simulink model "PMSM_Model"  (R2024b)
settings: Solver=FixedStepAuto  StartTime=0.0  StopTime=3  FixedStep=1e-5  MaxStep=1e-4  RelTol=1e-4
model workspace: external: MAT-File D:\EV\Graduation_project\Motor_Model_mathmatical\Model_Calculations.mat (data not in the file)
undefined symbols (not defined in the file): B, f, J, Ki_d, Ki_q, Ki_s, Kp_q, Kp_s, lambda, lamdaM, Ld, Ls, p, P, R, Rs, Tc, Vm
libraries: simulink x3, eeStairGenerator x1
settings Model: Creator=ahmed  LastModifiedBy=ahmed
settings SolverCC: ZeroCrossAlgorithm=Adaptive
settings DebuggingCC: ConsistencyChecking=warning  IgnoredZcDiagnostic=none

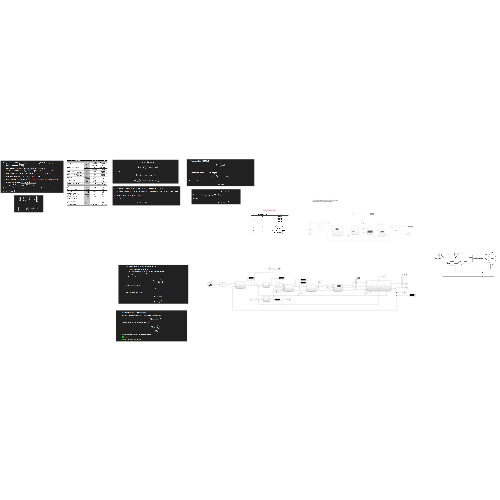
[thumbnail: Simulink's stored preview of the top-level diagram]
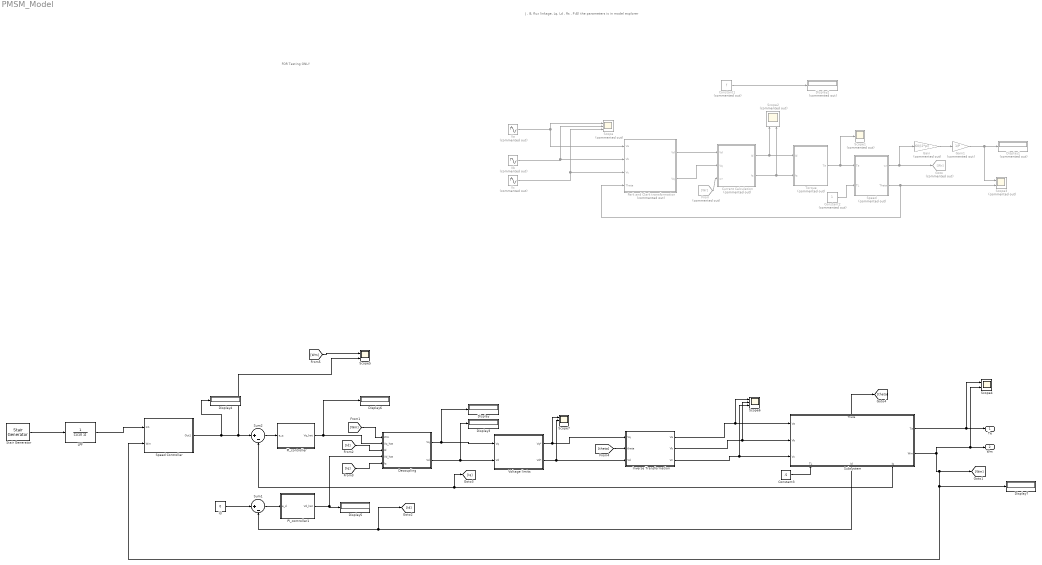
== system PMSM_Model ==
  note: FOR Testing ONLY
  note: J , B, flux linkage, Lq, Ld , Rs , P All the parameters is in model explorer
  Constant1 : Constant  Commented=on  Value=f
  Constant2 : Constant  Commented=on
  Constant3 : Constant  Value=.5
  Current Calculation : Subsystem  Commented=on
  "Decoupling " : Subsystem
  Display{,3..7} (6 alike) : Display
  Display1 : Display  Commented=on
  Display2 : Display  Commented=on
  From : From  Commented=on  GotoTag=Wr
  Gain : Gain  Commented=on  Gain=60/(2*pi)
  Gain1 : Gain  Commented=on  Gain=1/P
  Goto : Goto  Commented=on  GotoTag=Wr
  Id : Constant  Value=0
  Inverse Transformation : Subsystem
  LPF : TransferFcn  Denominator=[1/10 1]
  PI_controller : Subsystem
  PI_controller1 : Subsystem
  Park and Clark transformation : Subsystem  Commented=on
  Scope : Scope  Commented=on  NumInputPorts=3
  Scope1 : Scope  Commented=on
  Scope2 : Scope  Commented=on  NumInputPorts=2
  Scope3 : Scope  Commented=on  NumInputPorts=2
  Scope4 : Scope  NumInputPorts=2
  Scope5 : Scope  NumInputPorts=2
  Scope6 : Scope  NumInputPorts=3
  Scope7 : Scope  NumInputPorts=3
  Speed : Subsystem  Commented=on
  "Speed Controller " : Subsystem
  Stair Generator : eeStairGenerator/Stair Generator  LabelModeActiveChoice=Discrete  TimeInput=[0 1 1.3 1.7 2 2.4]  AmplitudeInput=[200 1000 3000 4500 2000 0]  SampleTime=1e-5  RepeatPattern=off  OutDataTypeStr=double
      settings: LibrarySourceBlock=ee_sl_lib/General Control/Stair Generator
  Subsystem : Subsystem
      settings: PortSchema="{\"entries\":[{\"content\":{\"sides\":[{\"content\":{\"connectorIds\":[\"In1\",\"In2\",\"In3\"]},\"type\":\"ConnectorPlacement.EquallySpacedRectSide\",\"uuid\":\"410fafe1-6d3d-4b62-9ccb-454f6008b81a\"},{\"content\":{\"connectorIds\":[\"Out1\",\"Out2\"],\"side\":\"RIGHT\"},\"type\":\"ConnectorPlacement.EquallySpacedRectSide\",\"uuid\":\"b4215a85-6f2a-4bbd-a305-1fa3c25faaac\"},{\"content\":{\"connectorIds\":[\"Out5\"],\"side\":\"TOP\"},\"type\":\"ConnectorPlacement.EquallySpacedRectSide\",\"uuid\":\"c3471a58-e27d-4fa8-ab5e-4301d929309b\"},{\"content\":{\"connectorIds\":[\"In4\",\"Out3\",\"Out4\"],\"side\":\"BOTTOM\"},\"type\":\"ConnectorPlacement.EquallySpacedRectSide\",\"uuid\":\"92e7eecc-1ce6-457d-b998-008a2505e29d\"}]},\"type\":\"ConnectorPlacement.EquallySpacedConnector\",\"uuid\":\"8b1e994c-6614-4fb4-bf28-22b9fb88c59f\"}],\"packageUris\":[\"http://schema.mathworks.com/mf0/Connector/R2020b\"],\"version\":\"1.0\"}"
  Sum1 : Sum  Inputs=|+-
  Sum2 : Sum  Inputs=|+-
  "Torque " : Subsystem  Commented=on
  Va : Sin  Commented=on  Amplitude=Vm  Frequency=2*f*pi  SampleTime=0
  Vb : Sin  Commented=on  Amplitude=Vm  Frequency=2*f*pi  Phase=-(120*(pi/180))  SampleTime=0
  Vc : Sin  Commented=on  Amplitude=Vm  Frequency=2*f*pi  Phase=-(240*(pi/180))  SampleTime=0
  Voltage limits : Subsystem
  Te : Outport
  Wm : Outport  Port=2
  wires:
  Va/1 -> Park and Clark transformation/1(Va), Scope/1
  Vb/1 -> Scope/2, Park and Clark transformation/2(Vb)
  Vc/1 -> Scope/3, Park and Clark transformation/3(Vc)
  Park and Clark transformation/1(Vd) -> Current Calculation/1(Vd)
  Park and Clark transformation/2(Vq) -> Current Calculation/2(Vq)
  "Torque "/1(Te) -> Scope1/1, Speed/1(Te)
  Speed/1(wr) -> Goto/1, Gain/1
  From/1 -> Current Calculation/3(wr)
  Current Calculation/2(Iq) -> "Torque "/2(Iq), Scope2/2
  Current Calculation/1(Id) -> "Torque "/1(Id), Scope2/1
  Speed/2(Theta) -> Park and Clark transformation/4(Theta), Scope3/2
  Gain/1 -> Gain1/1
  Gain1/1 -> Scope3/1, Display1/1
  Constant1/1 -> Display2/1
  Inverse Transformation/1(Va) -> Scope6/1, Subsystem/1(Va)
  Inverse Transformation/2(Vb) -> Scope6/2, Subsystem/2(Vb)
  Inverse Transformation/3(Vc) -> Subsystem/3(Vc), Scope6/3
  Subsystem/2(Wm) -> Scope4/2, Wm/1, Display7/1, "Speed Controller "/2(Wm), [Wm]
  Subsystem/1(Te) -> Scope4/1, Te/1
  Subsystem/4(Iq) -> [Iq], Sum2/2
  Id/1 -> Sum1/1
  Subsystem/3(Id) -> [Id], Sum1/2
  "Speed Controller "/1(Out1) -> Display4/1, Scope5/2, Sum2/1
  Sum2/1 -> PI_controller/1(e_q)
  Sum1/1 -> PI_controller1/1(e_d)
  PI_controller/1(Vq_hat) -> Display6/1, "Decoupling "/2(Vq_hat)
  PI_controller1/1(Vd_hat) -> "Decoupling "/4(Vd_hat), Display5/1
  "Decoupling "/1(Vq) -> Display/1, Voltage limits/1(Vq)
  "Decoupling "/2(Vd) -> Display3/1, Voltage limits/2(Vd)
  Voltage limits/1(Vq*) -> Scope7/1, Inverse Transformation/1(Vq)
  Voltage limits/2(Vd*) -> Scope7/2, Inverse Transformation/3(Vd)
  Stair Generator/1 -> LPF/1
  Constant2/1 -> Speed/2(TL)
  [Wm] -> "Decoupling "/1(Wm)
  [Id] -> "Decoupling "/3(Id)
  [Iq] -> "Decoupling "/5(Iq)
  Subsystem/5(Theta) -> [theta]
  [theta] -> Inverse Transformation/2(theta)
  Constant3/1 -> Subsystem/4(TL)
  [Wm] -> Scope5/1
  LPF/1 -> "Speed Controller "/1(In1)

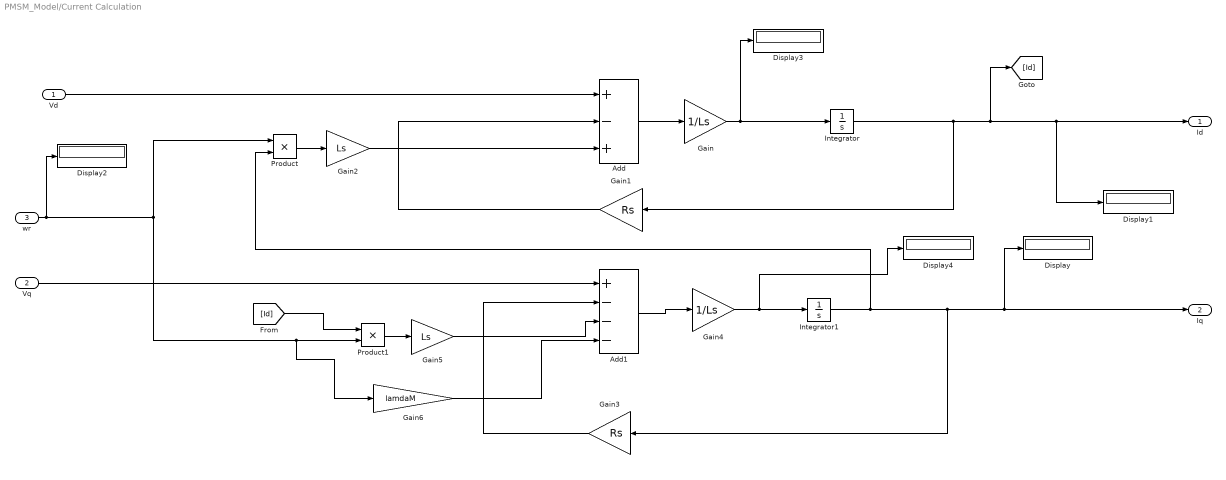
== system PMSM_Model/Current Calculation ==
  Vd : Inport
  Vq : Inport  Port=2
  wr : Inport  Port=3
  Add : Sum  Inputs=+-+
  Add1 : Sum  Inputs=+---
  Display{,1..4} (5 alike) : Display
  Gain : Gain  Gain=1/Ls
  Gain1 : Gain  Gain=Rs
  Gain2 : Gain  Gain=Ls
  Gain3 : Gain  Gain=Rs
  Gain4 : Gain  Gain=1/Ls
  Gain5 : Gain  Gain=Ls
  Gain6 : Gain  Gain=lamdaM
  Integrator : Integrator
  Integrator1 : Integrator
  Product : Product
  Product1 : Product
  Id : Outport
  Iq : Outport  Port=2
  wires:
  Vd/1 -> Add/1
  Add/1 -> Gain/1
  Gain/1 -> Integrator/1, Display3/1
  Integrator/1 -> Gain1/1, [Id], Display1/1, Id/1
  Gain1/1 -> Add/2
  wr/1 -> Product/1, Gain6/1, Product1/2, Display2/1
  Product/1 -> Gain2/1
  Gain2/1 -> Add/3
  Vq/1 -> Add1/1
  Add1/1 -> Gain4/1
  Gain4/1 -> Display4/1, Integrator1/1
  Integrator1/1 -> Product/2, Display/1, Iq/1, Gain3/1
  Gain3/1 -> Add1/2
  [Id] -> Product1/1
  Product1/1 -> Gain5/1
  Gain5/1 -> Add1/3
  Gain6/1 -> Add1/4

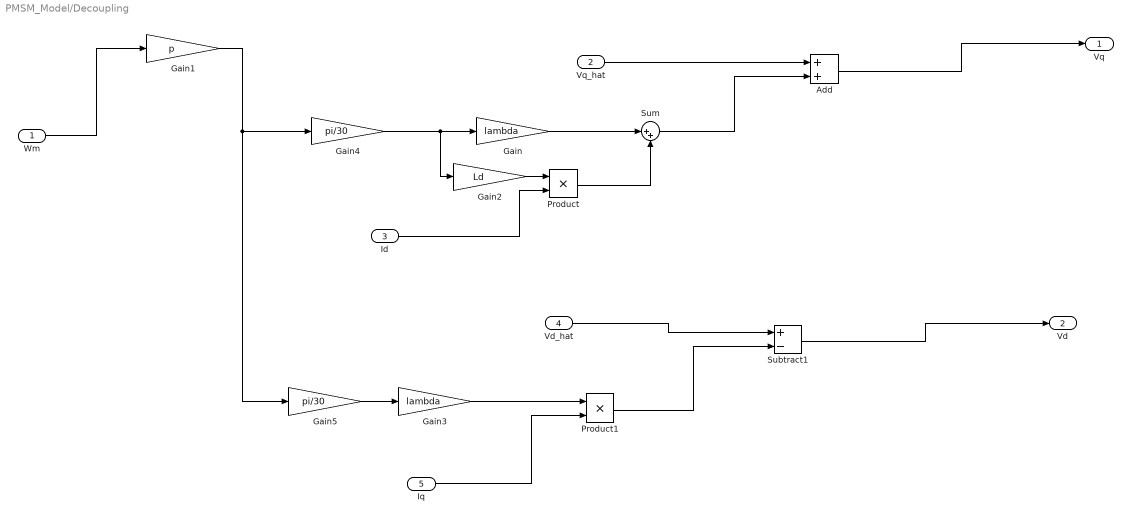
== system PMSM_Model/Decoupling  ==
  Wm : Inport
  Vq_hat : Inport  Port=2
  Id : Inport  Port=3
  Vd_hat : Inport  Port=4
  Iq : Inport  Port=5
  Add : Sum
  Gain : Gain  Gain=lambda
  Gain1 : Gain  Gain=p
  Gain2 : Gain  Gain=Ld
  Gain3 : Gain  Gain=lambda
  Gain4 : Gain  Gain=pi/30
  Gain5 : Gain  Gain=pi/30
  Product : Product
  Product1 : Product
  Subtract1 : Sum  Inputs=+-
  Sum : Sum  Inputs=|++
  Vq : Outport
  Vd : Outport  Port=2
  wires:
  Vq_hat/1 -> Add/1
  Vd_hat/1 -> Subtract1/1
  Wm/1 -> Gain1/1
  Gain1/1 -> Gain4/1, Gain5/1
  Gain2/1 -> Product/1
  Id/1 -> Product/2
  Product/1 -> Sum/2
  Gain/1 -> Sum/1
  Sum/1 -> Add/2
  Gain3/1 -> Product1/1
  Product1/1 -> Subtract1/2
  Iq/1 -> Product1/2
  Gain4/1 -> Gain2/1, Gain/1
  Add/1 -> Vq/1
  Subtract1/1 -> Vd/1
  Gain5/1 -> Gain3/1

== system PMSM_Model/Inverse Transformation ==
  Vq : Inport
  theta : Inport  Port=2
  Vd : Inport  Port=3
  "Inverse Park " : Subsystem
  inverse Clark : Subsystem
  Va : Outport
  Vb : Outport  Port=2
  Vc : Outport  Port=3
  wires:
  Vq/1 -> "Inverse Park "/3(In3)
  theta/1 -> "Inverse Park "/1(In1)
  Vd/1 -> "Inverse Park "/2(In2)
  "Inverse Park "/1(Valpha) -> inverse Clark/1(In1)
  "Inverse Park "/2(Vbeta) -> inverse Clark/2(In2)
  inverse Clark/1(Va) -> Va/1
  inverse Clark/2(Vb) -> Vb/1
  inverse Clark/3(Vc) -> Vc/1

== system PMSM_Model/PI_controller ==
  note: Kp = ((2*zeta*wn)-(Rs/ld))*Ld
  note: Kp = (Wn^2)*Ld
  e_q : Inport
  Display : Display
  Integrator : Integrator
  Ki : Gain  Gain=Ki_q
  Kp : Gain  Gain=Kp_q
  Product : Product
  Scope : Scope
  Sum : Sum  Inputs=|++
  Vq_hat : Outport
  wires:
  Kp/1 -> Sum/1
  Sum/1 -> Display/1, Vq_hat/1
  e_q/1 -> Ki/1, Kp/1
  [Stop_q_integrator] -> Scope/1, Product/2
  Product/1 -> Integrator/1
  Integrator/1 -> Sum/2
  Ki/1 -> Product/1

== system PMSM_Model/PI_controller1 ==
  e_d : Inport
  Integrator : Integrator
  Ki : Gain  Gain=Ki_d
  Kp : Gain  Gain=Kp_q
  Product : Product
  Sum : Sum  Inputs=|++
  Time Scope : Scope
  Vd_hat : Outport
  wires:
  Kp/1 -> Sum/1
  e_d/1 -> Ki/1, Kp/1
  Sum/1 -> Vd_hat/1
  Product/1 -> Integrator/1
  [Stop_d_integrator] -> Product/2, Time Scope/1
  Integrator/1 -> Sum/2
  Ki/1 -> Product/1

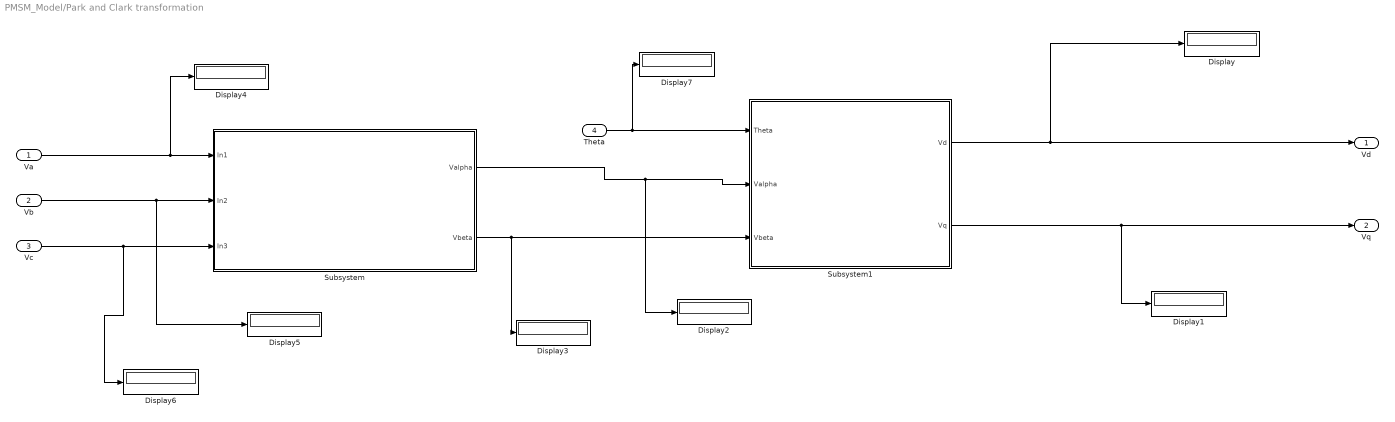
== system PMSM_Model/Park and Clark transformation ==
  Va : Inport
  Vb : Inport  Port=2
  Vc : Inport  Port=3
  Theta : Inport  Port=4
  Display{,1..7} (8 alike) : Display
  Subsystem : Subsystem
  Subsystem1 : Subsystem
  Vd : Outport
  Vq : Outport  Port=2
  wires:
  Va/1 -> Display4/1, Subsystem/1(In1)
  Vb/1 -> Display5/1, Subsystem/2(In2)
  Vc/1 -> Display6/1, Subsystem/3(In3)
  Subsystem/1(Valpha) -> Display2/1, Subsystem1/2(Valpha)
  Subsystem/2(Vbeta) -> Display3/1, Subsystem1/3(Vbeta)
  Subsystem1/1(Vd) -> Display/1, Vd/1
  Subsystem1/2(Vq) -> Vq/1, Display1/1
  Theta/1 -> Display7/1, Subsystem1/1(Theta)

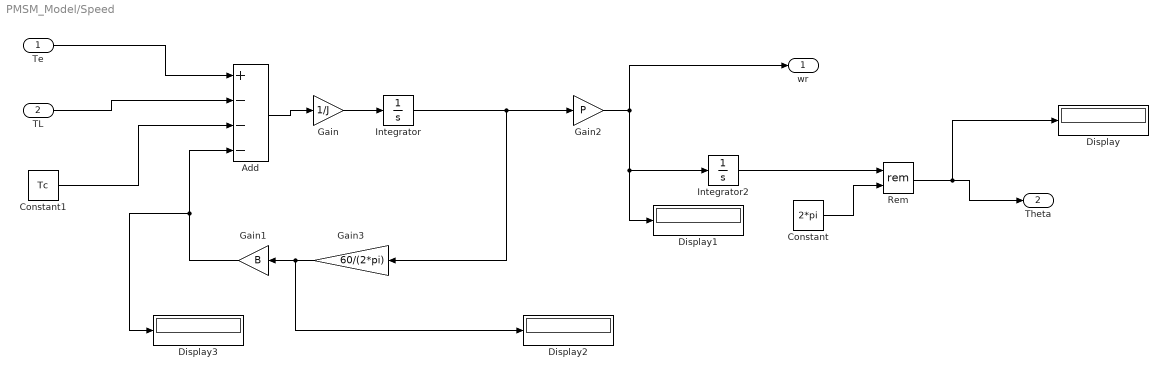
== system PMSM_Model/Speed ==
  Te : Inport
  TL : Inport  Port=2
  Add : Sum  Inputs=+---
  Constant : Constant  Value=2*pi
  Constant1 : Constant  Value=Tc
  Display{,1..3} (4 alike) : Display
  Gain : Gain  Gain=1/J
  Gain1 : Gain  Gain=B
  Gain2 : Gain  Gain=P
  Gain3 : Gain  Gain=60/(2*pi)
  Integrator : Integrator
  Integrator2 : Integrator
  Rem : Math  Operator=rem
  wr : Outport
  Theta : Outport  Port=2
  wires:
  Te/1 -> Add/1
  Gain/1 -> Integrator/1
  TL/1 -> Add/2
  Add/1 -> Gain/1
  Gain1/1 -> Display3/1, Add/4
  Integrator/1 -> Gain3/1, Gain2/1
  Gain2/1 -> Display1/1, Integrator2/1, wr/1
  Integrator2/1 -> Rem/1
  Constant/1 -> Rem/2
  Rem/1 -> Display/1, Theta/1
  Constant1/1 -> Add/3
  Gain3/1 -> Display2/1, Gain1/1

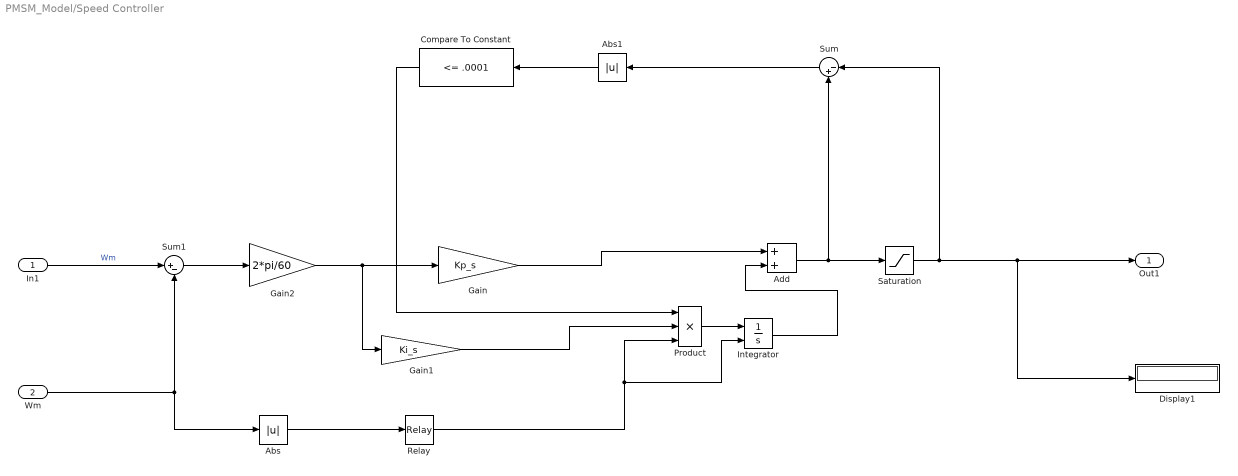
== system PMSM_Model/Speed Controller  ==
  In1 : Inport
  Wm : Inport  Port=2
  Abs : Abs  SaturateOnIntegerOverflow=off
  Abs1 : Abs  SaturateOnIntegerOverflow=off
  Add : Sum
  Compare To Constant : simulink/Logic and Bit Operations/Compare To Constant  relop=<=  const=.0001  OutDataTypeStr=boolean
  Display1 : Display
  Gain : Gain  Gain=Kp_s
  Gain1 : Gain  Gain=Ki_s
  Gain2 : Gain  Gain=2*pi/60
  Integrator : Integrator  ExternalReset=falling
  Product : Product  Inputs=3
  Relay : Relay  OnSwitchValue=100  OffSwitchValue=-100
  Saturation : Saturate  UpperLimit=12  LowerLimit=-12
  Sum : Sum  Inputs=|-+
  Sum1 : Sum  Inputs=|+-
  Out1 : Outport
  wires:
  Gain/1 -> Add/1
  Add/1 -> Saturation/1, Sum/2
  Gain2/1 -> Gain/1, Gain1/1
  In1/1 -> Sum1/1  "Wm"
  Wm/1 -> Abs/1, Sum1/2
  Sum1/1 -> Gain2/1
  Abs/1 -> Relay/1
  Product/1 -> Integrator/1
  Saturation/1 -> Sum/1, Out1/1, Display1/1
  Abs1/1 -> Compare To Constant/1
  Sum/1 -> Abs1/1
  Compare To Constant/1 -> Product/1
  Gain1/1 -> Product/2
  Relay/1 -> Integrator/2, Product/3
  Integrator/1 -> Add/2

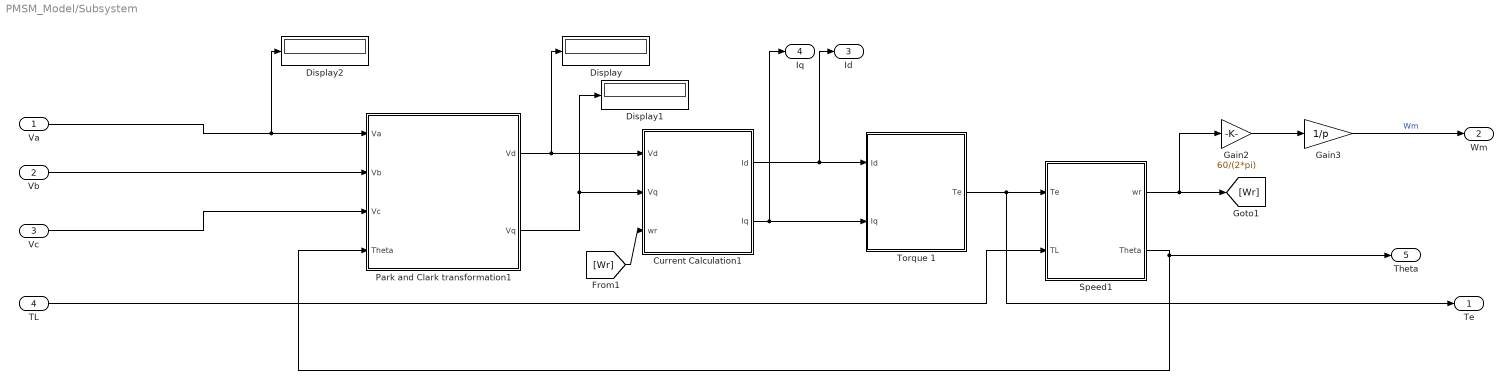
== system PMSM_Model/Subsystem ==
  Va : Inport
  Vb : Inport  Port=2
  Vc : Inport  Port=3
  TL : Inport  Port=4
  Current Calculation1 : Subsystem
  Display : Display
  Display1 : Display
  Display2 : Display
  Gain2 : Gain  Gain=60/(2*pi)
  Gain3 : Gain  Gain=1/p
  Park and Clark transformation1 : Subsystem
  Speed1 : Subsystem
  Torque 1 : Subsystem
  Te : Outport
  Wm : Outport  Port=2
  Id : Outport  Port=3
  Iq : Outport  Port=4
  Theta : Outport  Port=5
  wires:
  [Wr] -> Current Calculation1/3(wr)
  Va/1 -> Display2/1, Park and Clark transformation1/1(Va)
  Park and Clark transformation1/2(Vq) -> Current Calculation1/2(Vq), Display1/1
  Torque 1/1(Te) -> Te/1, Speed1/1(Te)
  Speed1/1(wr) -> Gain2/1, [Wr]
  Park and Clark transformation1/1(Vd) -> Display/1, Current Calculation1/1(Vd)
  Gain2/1 -> Gain3/1
  Speed1/2(Theta) -> Park and Clark transformation1/4(Theta), Theta/1
  Current Calculation1/2(Iq) -> Torque 1/2(Iq), Iq/1
  Current Calculation1/1(Id) -> Id/1, Torque 1/1(Id)
  Vb/1 -> Park and Clark transformation1/2(Vb)
  Gain3/1 -> Wm/1  "Wm"
  Vc/1 -> Park and Clark transformation1/3(Vc)
  TL/1 -> Speed1/2(TL)

== system PMSM_Model/Torque  ==
  Id : Inport
  Iq : Inport  Port=2
  Display : Display
  Display1 : Display
  Gain : Gain  Gain=lamdaM
  Gain1 : Gain  Gain=P
  Gain2 : Gain  Gain=3/2
  Gain3 : Gain
  Te : Outport
  wires:
  Iq/1 -> Display1/1, Gain/1
  Gain/1 -> Gain1/1
  Gain2/1 -> Display/1, Gain3/1
  Gain1/1 -> Gain2/1
  Gain3/1 -> Te/1

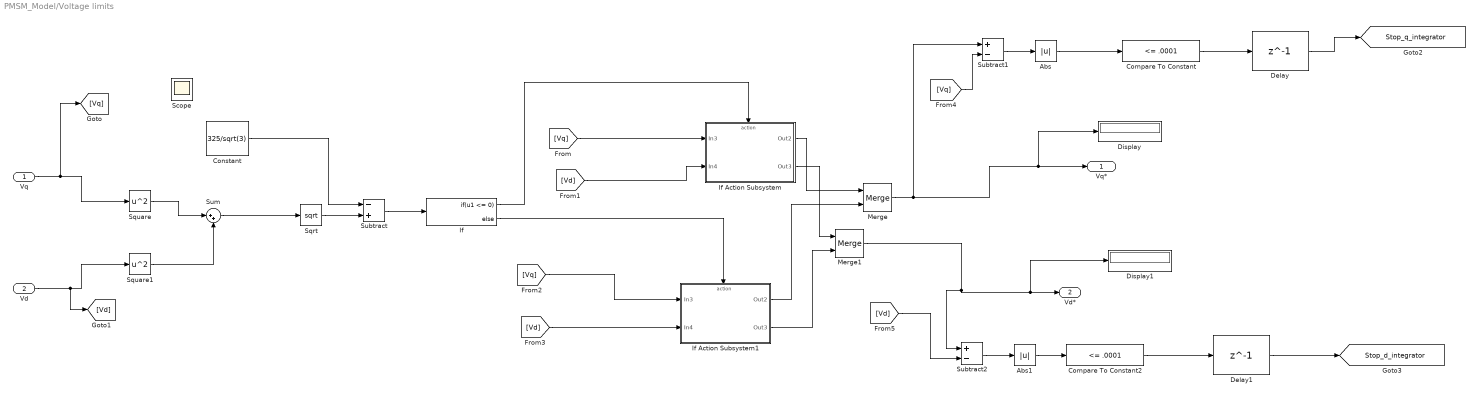
== system PMSM_Model/Voltage limits ==
  Vq : Inport
  Vd : Inport  Port=2
  Abs : Abs  SaturateOnIntegerOverflow=off
  Abs1 : Abs  SaturateOnIntegerOverflow=off
  Compare To Constant : simulink/Logic and Bit Operations/Compare To Constant  relop=<=  const=.0001  OutDataTypeStr=boolean
  Compare To Constant2 : simulink/Logic and Bit Operations/Compare To Constant  relop=<=  const=.0001  OutDataTypeStr=boolean
  Constant : Constant  Value=325/sqrt(3)
  Delay : Delay  DelayLength=1
  Delay1 : Delay  DelayLength=1
  Display : Display
  Display1 : Display
  If : If  IfExpression=u1 <= 0
  If Action Subsystem : Subsystem  TreatAsAtomicUnit=on
  If Action Subsystem1 : Subsystem  TreatAsAtomicUnit=on
  Merge : Merge
  Merge1 : Merge
  Scope : Scope
  Sqrt : Sqrt
  Square : Math  Operator=square
  Square1 : Math  Operator=square
  Subtract : Sum  Inputs=-+
  Subtract1 : Sum  Inputs=+-
  Subtract2 : Sum  Inputs=+-
  Sum : Sum  Inputs=|++
  Vq* : Outport
  Vd* : Outport  Port=2
  tag scope: Stop_d_integrator=global, Stop_q_integrator=global
  wires:
  Vq/1 -> [Vq], Square/1
  Vd/1 -> [Vd], Square1/1
  Square/1 -> Sum/1
  Square1/1 -> Sum/2
  Sum/1 -> Sqrt/1
  Sqrt/1 -> Subtract/2
  Constant/1 -> Subtract/1
  Subtract/1 -> If/1
  If/1 -> If Action Subsystem/Action
  If/2 -> If Action Subsystem1/Action
  [Vq] -> If Action Subsystem/1(In3)
  [Vd] -> If Action Subsystem/2(In4)
  [Vq] -> If Action Subsystem1/1(In3)
  [Vd] -> If Action Subsystem1/2(In4)
  If Action Subsystem/1(Out2) -> Merge/1
  If Action Subsystem1/1(Out2) -> Merge/2
  If Action Subsystem/2(Out3) -> Merge1/1
  If Action Subsystem1/2(Out3) -> Merge1/2
  Merge/1 -> Display/1, Vq*/1, Subtract1/1
  [Vq] -> Subtract1/2
  Subtract1/1 -> Abs/1
  Abs/1 -> Compare To Constant/1
  Abs1/1 -> Compare To Constant2/1
  Subtract2/1 -> Abs1/1
  [Vd] -> Subtract2/2
  Compare To Constant/1 -> Delay/1
  Compare To Constant2/1 -> Delay1/1
  Delay/1 -> [Stop_q_integrator]
  Delay1/1 -> [Stop_d_integrator]
  Merge1/1 -> Subtract2/1, Display1/1, Vd*/1

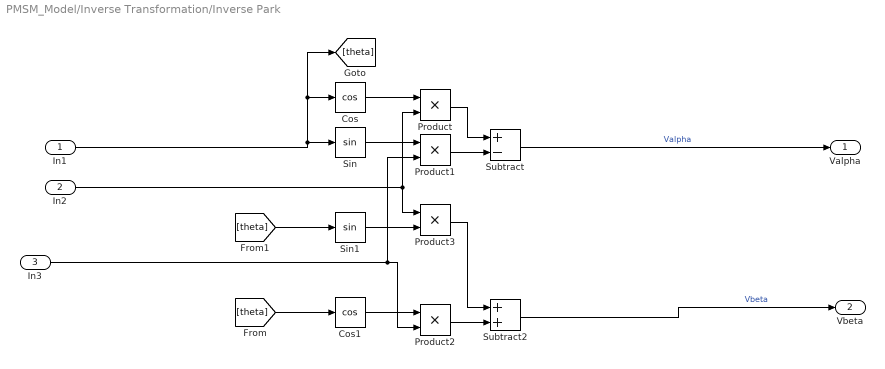
== system PMSM_Model/Inverse Transformation/Inverse Park  ==
  In1 : Inport
  In2 : Inport  Port=2
  In3 : Inport  Port=3
  Cos : Trigonometry  Operator=cos
  Cos1 : Trigonometry  Operator=cos
  Product{,1..3} (4 alike) : Product
  Sin : Trigonometry
  Sin1 : Trigonometry
  Subtract : Sum  Inputs=+-
  Subtract2 : Sum
  Valpha : Outport
  Vbeta : Outport  Port=2
  wires:
  Product3/1 -> Subtract2/1
  In3/1 -> Product2/2, Product1/2
  In1/1 -> Cos/1, [theta], Sin/1
  Subtract/1 -> Valpha/1  "Valpha"
  Product/1 -> Subtract/1
  Subtract2/1 -> Vbeta/1  "Vbeta"
  Product2/1 -> Subtract2/2
  Cos/1 -> Product/1
  Product1/1 -> Subtract/2
  [theta] -> Cos1/1
  In2/1 -> Product/2, Product3/1
  [theta] -> Sin1/1
  Sin/1 -> Product1/1
  Cos1/1 -> Product2/1
  Sin1/1 -> Product3/2

== system PMSM_Model/Inverse Transformation/inverse Clark ==
  In1 : Inport
  In2 : Inport  Port=2
  Add : Sum
  Add1 : Sum
  Constant : Constant  Value=-1/2
  Constant1 : Constant  Value=sqrt(3)/2
  Constant2 : Constant  Value=-1/2
  Constant3 : Constant  Value=-sqrt(3)/2
  Product{,1..3} (4 alike) : Product
  Va : Outport
  Vb : Outport  Port=2
  Vc : Outport  Port=3
  wires:
  In1/1 -> Va/1, Product1/2, Product2/2
  In2/1 -> Product/1, Product3/2
  Add/1 -> Vb/1
  Product3/1 -> Add1/2
  Constant/1 -> Product1/1
  Constant2/1 -> Product2/1
  Product/1 -> Add/2
  Constant1/1 -> Product/2
  Product1/1 -> Add/1
  Product2/1 -> Add1/1
  Add1/1 -> Vc/1
  Constant3/1 -> Product3/1

== system PMSM_Model/Park and Clark transformation/Subsystem ==
  In1 : Inport
  In2 : Inport  Port=2
  In3 : Inport  Port=3
  Add : Sum  Inputs=+--
  Add1 : Sum  Inputs=+-
  Gain : Gain  Gain=2/3
  Gain1 : Gain  Gain=1/2
  Gain2 : Gain  Gain=1/2
  Gain3 : Gain  Gain=sqrt(3)/2
  Gain4 : Gain  Gain=sqrt(3)/2
  Gain5 : Gain  Gain=2/3
  Valpha : Outport
  Vbeta : Outport  Port=2
  wires:
  Gain3/1 -> Add1/1
  Gain1/1 -> Add/3
  Gain2/1 -> Add/2
  In2/1 -> Gain2/1, Gain3/1
  Gain5/1 -> Vbeta/1
  Gain4/1 -> Add1/2
  In3/1 -> Gain1/1, Gain4/1
  Add/1 -> Gain/1
  Add1/1 -> Gain5/1
  Gain/1 -> Valpha/1
  In1/1 -> Add/1

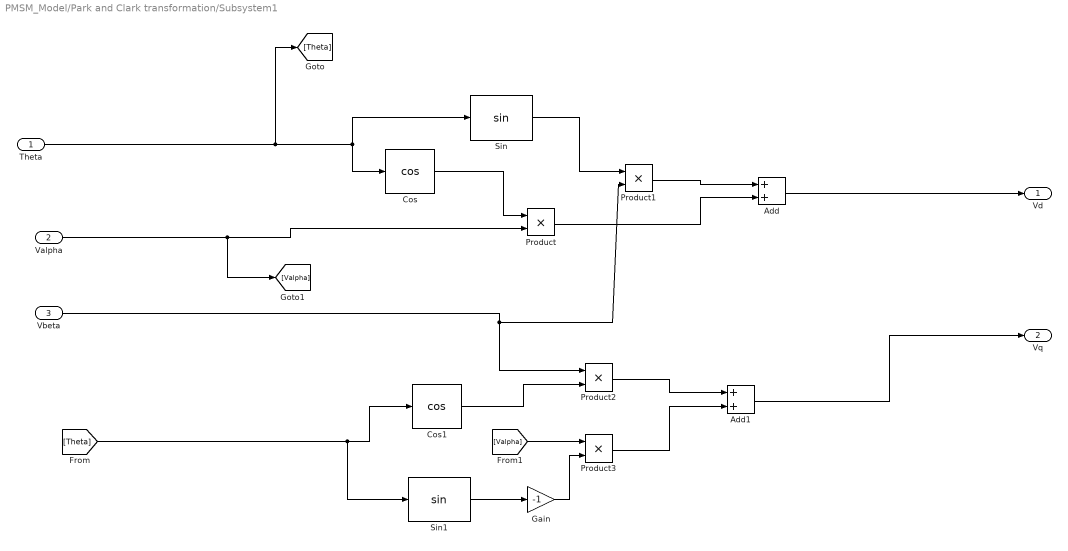
== system PMSM_Model/Park and Clark transformation/Subsystem1 ==
  Theta : Inport
  Valpha : Inport  Port=2
  Vbeta : Inport  Port=3
  Add : Sum
  Add1 : Sum
  Cos : Trigonometry  Operator=cos
  Cos1 : Trigonometry  Operator=cos
  Gain : Gain  Gain=-1
  Product{,1..3} (4 alike) : Product
  Sin : Trigonometry
  Sin1 : Trigonometry
  Vd : Outport
  Vq : Outport  Port=2
  wires:
  Sin1/1 -> Gain/1
  Gain/1 -> Product3/2
  Product/1 -> Add/2
  Sin/1 -> Product1/1
  Theta/1 -> [Theta], Cos/1, Sin/1
  Product1/1 -> Add/1
  [Theta] -> Sin1/1, Cos1/1
  Cos1/1 -> Product2/2
  Cos/1 -> Product/1
  Product3/1 -> Add1/2
  Product2/1 -> Add1/1
  Vbeta/1 -> Product2/1, Product1/2
  [Valpha] -> Product3/1
  Add/1 -> Vd/1
  Valpha/1 -> [Valpha], Product/2
  Add1/1 -> Vq/1

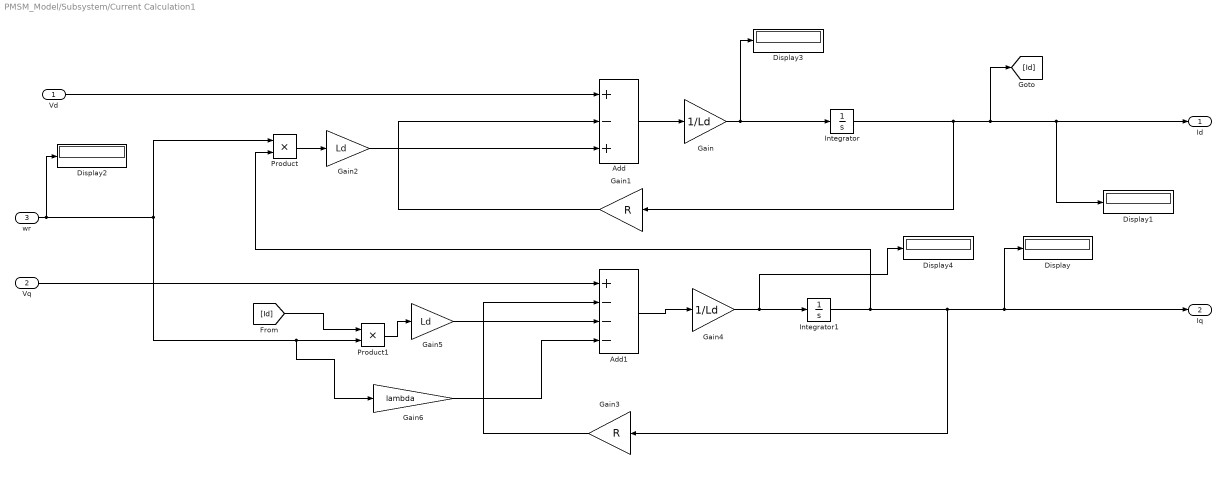
== system PMSM_Model/Subsystem/Current Calculation1 ==
  Vd : Inport
  Vq : Inport  Port=2
  wr : Inport  Port=3
  Add : Sum  Inputs=+-+
  Add1 : Sum  Inputs=+---
  Display{,1..4} (5 alike) : Display
  Gain : Gain  Gain=1/Ld
  Gain1 : Gain  Gain=R
  Gain2 : Gain  Gain=Ld
  Gain3 : Gain  Gain=R
  Gain4 : Gain  Gain=1/Ld
  Gain5 : Gain  Gain=Ld
  Gain6 : Gain  Gain=lambda
  Integrator : Integrator
  Integrator1 : Integrator
  Product : Product
  Product1 : Product
  Id : Outport
  Iq : Outport  Port=2
  wires:
  Gain6/1 -> Add1/4
  Gain5/1 -> Add1/3
  Product1/1 -> Gain5/1
  [Id] -> Product1/1
  Gain3/1 -> Add1/2
  Integrator1/1 -> Gain3/1, Iq/1, Display/1, Product/2
  Gain4/1 -> Integrator1/1, Display4/1
  Add1/1 -> Gain4/1
  Vq/1 -> Add1/1
  Gain2/1 -> Add/3
  Product/1 -> Gain2/1
  wr/1 -> Display2/1, Product1/2, Gain6/1, Product/1
  Gain1/1 -> Add/2
  Integrator/1 -> Id/1, Display1/1, [Id], Gain1/1
  Gain/1 -> Display3/1, Integrator/1
  Add/1 -> Gain/1
  Vd/1 -> Add/1

== system PMSM_Model/Subsystem/Park and Clark transformation1 ==
  Va : Inport
  Vb : Inport  Port=2
  Vc : Inport  Port=3
  Theta : Inport  Port=4
  Display{,1..7} (8 alike) : Display
  Subsystem : Subsystem
  Subsystem1 : Subsystem
  Vd : Outport
  Vq : Outport  Port=2
  wires:
  Theta/1 -> Subsystem1/1(Theta), Display7/1
  Subsystem1/2(Vq) -> Display1/1, Vq/1
  Subsystem1/1(Vd) -> Vd/1, Display/1
  Subsystem/2(Vbeta) -> Subsystem1/3(Vbeta), Display3/1
  Subsystem/1(Valpha) -> Subsystem1/2(Valpha), Display2/1
  Vc/1 -> Subsystem/3(In3), Display6/1
  Vb/1 -> Subsystem/2(In2), Display5/1
  Va/1 -> Subsystem/1(In1), Display4/1

== system PMSM_Model/Subsystem/Speed1 ==
  Te : Inport
  TL : Inport  Port=2
  Add : Sum  Inputs=+---
  Constant : Constant  Value=2*pi
  Constant1 : Constant  Value=.03
  Display : Display
  Display1 : Display
  Gain : Gain  Gain=1/J
  Gain1 : Gain  Gain=B
  Gain2 : Gain  Gain=p
  Integrator : Integrator
  Integrator2 : Integrator
  Rem : Math  Operator=rem
  wr : Outport
  Theta : Outport  Port=2
  wires:
  Constant1/1 -> Add/3
  Rem/1 -> Theta/1, Display/1
  Constant/1 -> Rem/2
  Integrator2/1 -> Rem/1
  Gain2/1 -> wr/1, Integrator2/1, Display1/1
  Gain1/1 -> Add/4
  Add/1 -> Gain/1
  TL/1 -> Add/2
  Gain/1 -> Integrator/1
  Te/1 -> Add/1
  Integrator/1 -> Gain1/1, Gain2/1

== system PMSM_Model/Subsystem/Torque 1 ==
  Id : Inport
  Iq : Inport  Port=2
  Display : Display
  Display1 : Display
  Gain : Gain  Gain=lambda
  Gain1 : Gain  Gain=p
  Gain2 : Gain  Gain=3/2
  Gain3 : Gain
  Saturation : Saturate  UpperLimit=3.82  LowerLimit=-3.82
  Te : Outport
  wires:
  Gain3/1 -> Te/1
  Gain1/1 -> Gain2/1
  Gain2/1 -> Saturation/1
  Gain/1 -> Gain1/1
  Iq/1 -> Gain/1, Display1/1
  Saturation/1 -> Gain3/1, Display/1

== system PMSM_Model/Voltage limits/If Action Subsystem ==
  In3 : Inport
  In4 : Inport  Port=2
  Action Port : ActionPort  ActionPortLabel=if(u1 <= 0)
  Cast To Single : DataTypeConversion  OutDataTypeStr=single  SaturateOnIntegerOverflow=off  RndMeth=Floor
  Cast To Single1 : DataTypeConversion  OutDataTypeStr=single  SaturateOnIntegerOverflow=off  RndMeth=Floor
  Out2 : Outport
  Out3 : Outport  Port=2
  wires:
  In3/1 -> Cast To Single/1
  In4/1 -> Cast To Single1/1
  Cast To Single/1 -> Out2/1
  Cast To Single1/1 -> Out3/1

== system PMSM_Model/Voltage limits/If Action Subsystem1 ==
  In3 : Inport
  In4 : Inport  Port=2
  Action Port : ActionPort  ActionPortLabel=else
  Divide1 : Product  Inputs=*/  OutDataTypeStr=single
  Divide2 : Product  Inputs=/*  OutDataTypeStr=single
  Gain : Gain  Gain=sqrt(3)
  Gain1 : Gain  Gain=325 * .95
  Gain2 : Gain  Gain=325 * .95
  Square : Math  Operator=square  OutDataTypeStr=single
  Square Root : Sqrt  OutDataTypeStr=single  IntermediateResultsDataTypeStr=single
  Square1 : Math  Operator=square  OutDataTypeStr=single
  Sum : Sum  OutDataTypeStr=single  AccumDataTypeStr=single
  Out2 : Outport
  Out3 : Outport  Port=2
  wires:
  Divide1/1 -> Out2/1
  Divide2/1 -> Out3/1
  Square/1 -> Sum/1
  Sum/1 -> Square Root/1
  In3/1 -> Square/1, Gain1/1
  Gain2/1 -> Divide2/2
  Square1/1 -> Sum/2
  Square Root/1 -> Gain/1
  In4/1 -> Square1/1, Gain2/1
  Gain1/1 -> Divide1/1
  Gain/1 -> Divide2/1, Divide1/2

== system PMSM_Model/Subsystem/Park and Clark transformation1/Subsystem ==
  In1 : Inport
  In2 : Inport  Port=2
  In3 : Inport  Port=3
  Add : Sum  Inputs=+--
  Add1 : Sum  Inputs=+-
  Gain : Gain  Gain=2/3
  Gain1 : Gain  Gain=1/2
  Gain2 : Gain  Gain=1/2
  Gain3 : Gain  Gain=sqrt(3)/2
  Gain4 : Gain  Gain=sqrt(3)/2
  Gain5 : Gain  Gain=2/3
  Valpha : Outport
  Vbeta : Outport  Port=2
  wires:
  In1/1 -> Add/1
  Gain/1 -> Valpha/1
  Add1/1 -> Gain5/1
  Add/1 -> Gain/1
  In3/1 -> Gain4/1, Gain1/1
  Gain4/1 -> Add1/2
  Gain5/1 -> Vbeta/1
  In2/1 -> Gain3/1, Gain2/1
  Gain2/1 -> Add/2
  Gain1/1 -> Add/3
  Gain3/1 -> Add1/1

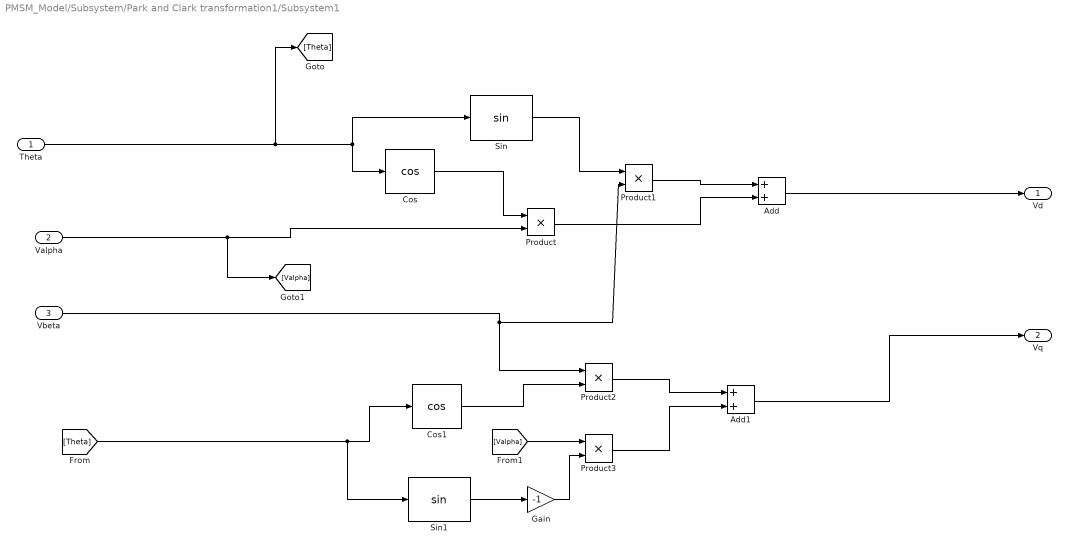
== system PMSM_Model/Subsystem/Park and Clark transformation1/Subsystem1 ==
  Theta : Inport
  Valpha : Inport  Port=2
  Vbeta : Inport  Port=3
  Add : Sum
  Add1 : Sum
  Cos : Trigonometry  Operator=cos
  Cos1 : Trigonometry  Operator=cos
  Gain : Gain  Gain=-1
  Product{,1..3} (4 alike) : Product
  Sin : Trigonometry
  Sin1 : Trigonometry
  Vd : Outport
  Vq : Outport  Port=2
  wires:
  Add1/1 -> Vq/1
  Valpha/1 -> Product/2, [Valpha]
  Add/1 -> Vd/1
  [Valpha] -> Product3/1
  Vbeta/1 -> Product1/2, Product2/1
  Product2/1 -> Add1/1
  Product3/1 -> Add1/2
  Cos/1 -> Product/1
  Cos1/1 -> Product2/2
  [Theta] -> Cos1/1, Sin1/1
  Product1/1 -> Add/1
  Theta/1 -> Sin/1, Cos/1, [Theta]
  Sin/1 -> Product1/1
  Product/1 -> Add/2
  Gain/1 -> Product3/2
  Sin1/1 -> Gain/1
